simulink model "matrice_jacobienne"  (R2022b)
settings: Solver=VariableStepAuto  StartTime=0.0  StopTime=10.0  RelTol=1e-3
undefined symbols (not defined in the file): l1, l2
settings Model: Creator=cheye  LastModifiedBy=cheye

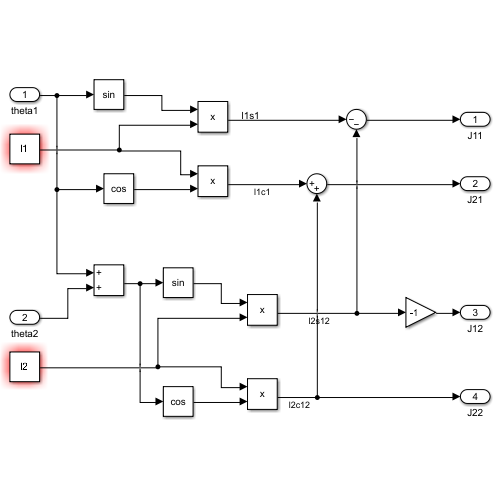
[thumbnail: Simulink's stored preview of the top-level diagram]
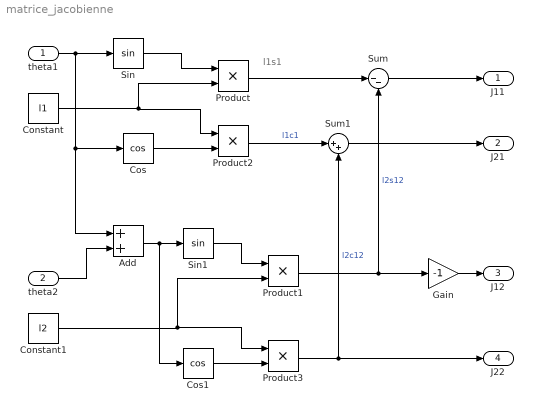
== system matrice_jacobienne ==
  note: l1s1
  theta1 : Inport
  theta2 : Inport  Port=2
  Add : Sum
  Constant : Constant  Value=l1
  Constant1 : Constant  Value=l2
  Cos : Trigonometry  Operator=cos
  Cos1 : Trigonometry  Operator=cos
  Gain : Gain  Gain=-1
  Product{,1..3} (4 alike) : Product
  Sin : Trigonometry
  Sin1 : Trigonometry
  Sum : Sum  Inputs=|--
  Sum1 : Sum  Inputs=|++
  J11 : Outport
  J21 : Outport  Port=2
  J12 : Outport  Port=3
  J22 : Outport  Port=4
  wires:
  Gain/1 -> J12/1
  Sum1/1 -> J21/1
  theta1/1 -> Cos/1, Add/1, Sin/1
  Product2/1 -> Sum1/1  "l1c1"
  Product1/1 -> Sum/2, Gain/1  "l2s12"
  theta2/1 -> Add/2
  Constant1/1 -> Product3/1, Product1/2
  Sum/1 -> J11/1
  Sin1/1 -> Product1/1
  Sin/1 -> Product/1
  Cos1/1 -> Product3/2
  Add/1 -> Cos1/1, Sin1/1
  Constant/1 -> Product/2, Product2/1
  Product/1 -> Sum/1
  Cos/1 -> Product2/2
  Product3/1 -> Sum1/2, J22/1  "l2c12"
